simulink model "fxpdemo_fix2fix"  (Simulink 7.6)
settings: Solver=FixedStepDiscrete  SolverMode=SingleTasking  StartTime=0.0  StopTime=0.9985  FixedStep=0.001  RelTol=1e-3  AbsTol=1e-6
Description:
  | Fixed-Point to Fixed-Point Conversion
  | 
  | An illustration of how to convert from fixed-point data type to another fixed-point datatype.
  | In this case the conversion is between sfix32_En2 and ufix8_En1, meaning:
  | 
  | * a signed 32-bit quantity with 2 bits to the right of the binary point
  | * an unsigned 8-bit quantity with 1 bit to the right of the binary point
settings Model: MinMaxOverflowLogging=MinMaxAndOverflow  Creator=The MathWorks Inc.  CovMetricSettings=d  ExtModeTrigMode=oneshot  ExtModeArmWhenConnect=off  ExtModeAutoUpdateStatusClock=off
settings DataIOCC: LimitDataPoints=off  SignalLoggingName=sigsOut
settings OptimizationCC: BooleanDataType=off  InlineInvariantSignals=on  InitFltsAndDblsToZero=on
settings DebuggingCC: SaveWithParameterizedLinksMsg=none  SignalResolutionControl=TryResolveAllWithWarning  SolverPrmCheckMsg=none  MultiTaskDSMMsg=warning  MultiTaskCondExecSysMsg=none  IntegerOverflowMsg=none  ParameterDowncastMsg=warning  ParameterOverflowMsg=warning  ParameterPrecisionLossMsg=none  StrictBusMsg=None
settings HardwareCC: TargetUnknown=on
settings RTWCC: IncludeERTFirstTime=on
settings GRTTargetCC: TargetFcnLib=ansi_tfl_tmw.mat

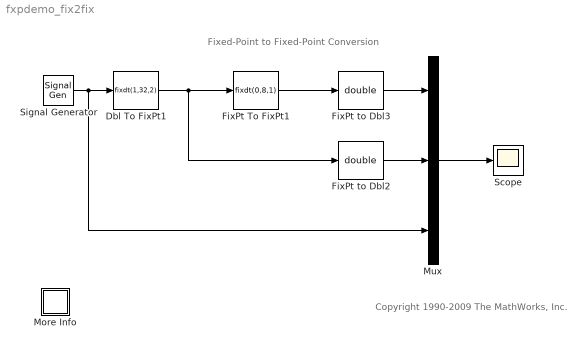
== system fxpdemo_fix2fix ==
  note: Copyright 1990-2009 The MathWorks, Inc.
  note: Fixed-Point to Fixed-Point Conversion
  Dbl To FixPt1 : DataTypeConversion  OutDataTypeStr=fixdt(1,32,2)  RndMeth=Nearest  SaturateOnIntegerOverflow=on
  FixPt To FixPt1 : DataTypeConversion  OutDataTypeStr=fixdt(0,8,1)  SaturateOnIntegerOverflow=on
  FixPt to Dbl2 : DataTypeConversion  OutDataTypeStr=double
  FixPt to Dbl3 : DataTypeConversion  OutDataTypeStr=double
  More Info : Subsystem
      settings: OpenFcn=showdemo(bdroot(gcs))
      mask Display: disp('?')
  Mux : Mux  Inputs=3
  Scope : Scope
      settings: TickLabels=on
  Signal Generator : SignalGenerator  WaveForm=sawtooth  Amplitude=5
  wires:
  Signal Generator/1 -> Dbl To FixPt1/1, Mux/3
  FixPt To FixPt1/1 -> FixPt to Dbl3/1
  FixPt to Dbl2/1 -> Mux/2
  FixPt to Dbl3/1 -> Mux/1
  Dbl To FixPt1/1 -> FixPt To FixPt1/1, FixPt to Dbl2/1
  Mux/1 -> Scope/1

== system fxpdemo_fix2fix/More Info ==
